simulink model "LQG_non_linear"  (R2022b)
settings: Solver=VariableStepAuto  StartTime=0.0  StopTime=100.0  RelTol=1e-3
values from neighbouring files (symbols this model uses):
  J = get_linearization()    [DK_iteration.m]    (also in LQG.m)
  Kr = lqr(J.A,J.B,Q,R)    [LQG.m]
undefined symbols (not defined in the file or in its folder): a, b, IPy, IPz, Ke, L, rp, std_dev_dx, std_dev_dy, std_dev_phi_dot, std_dev_psi
libraries: simulink x2
settings Model: Creator=alexi  LastModifiedBy=franc

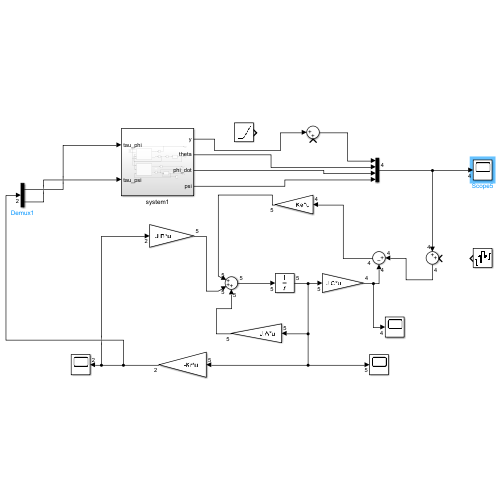
[thumbnail: Simulink's stored preview of the top-level diagram]
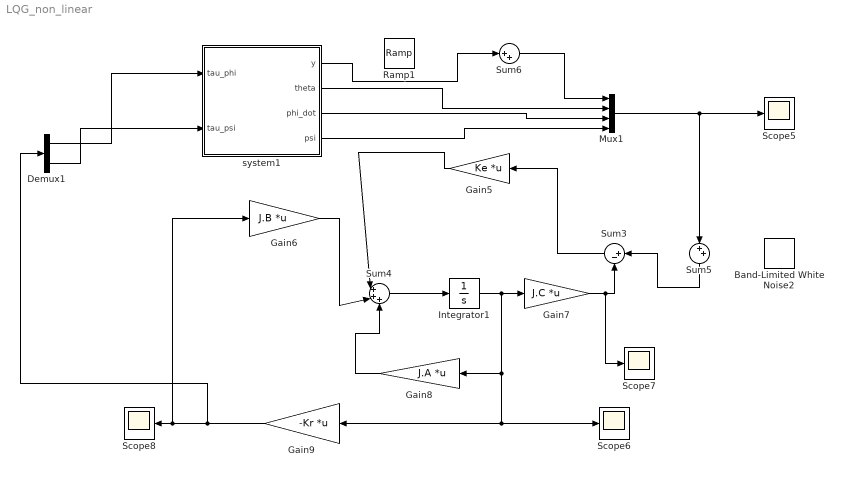
== system LQG_non_linear ==
  Band-Limited White Noise2 : simulink/Sources/Band-Limited White Noise  Cov=[std_dev_dx; std_dev_dy; std_dev_phi_dot; std_dev_psi]  Ts=0.1  seed=[23341]
  Demux1 : Demux  Outputs=2
  Gain5 : Gain  Gain=Ke  Multiplication=Matrix(K*u)
  Gain6 : Gain  Gain=J.B  Multiplication=Matrix(K*u)
  Gain7 : Gain  Gain=J.C  Multiplication=Matrix(K*u)
  Gain8 : Gain  Gain=J.A  Multiplication=Matrix(K*u)
  Gain9 : Gain  Gain=-Kr  Multiplication=Matrix(K*u)
  Integrator1 : Integrator
  Mux1 : Mux
  Ramp1 : simulink/Sources/Ramp  slope=1  start=0  InitialOutput=0
  Scope{5..8} (4 alike) : Scope
  Sum3 : Sum  Inputs=|+-
  Sum4 : Sum  Inputs=|+++
  Sum5 : Sum  Inputs=|++
  Sum6 : Sum  Inputs=|++
  system1 : Subsystem
  wires:
  Gain8/1 -> Sum4/3
  Mux1/1 -> Scope5/1, Sum5/1
  Sum6/1 -> Mux1/1
  Gain5/1 -> Sum4/1
  Gain7/1 -> Scope7/1, Sum3/2
  Sum4/1 -> Integrator1/1
  system1/2(theta) -> Mux1/2
  Sum5/1 -> Sum3/1
  Gain6/1 -> Sum4/2
  Integrator1/1 -> Scope6/1, Gain9/1, Gain8/1, Gain7/1
  Sum3/1 -> Gain5/1
  system1/1(y) -> Sum6/1
  system1/3(phi_dot) -> Mux1/3
  system1/4(psi) -> Mux1/4
  Gain9/1 -> Demux1/1, Gain6/1, Scope8/1
  Demux1/1 -> system1/1(tau_phi)
  Demux1/2 -> system1/2(tau_psi)

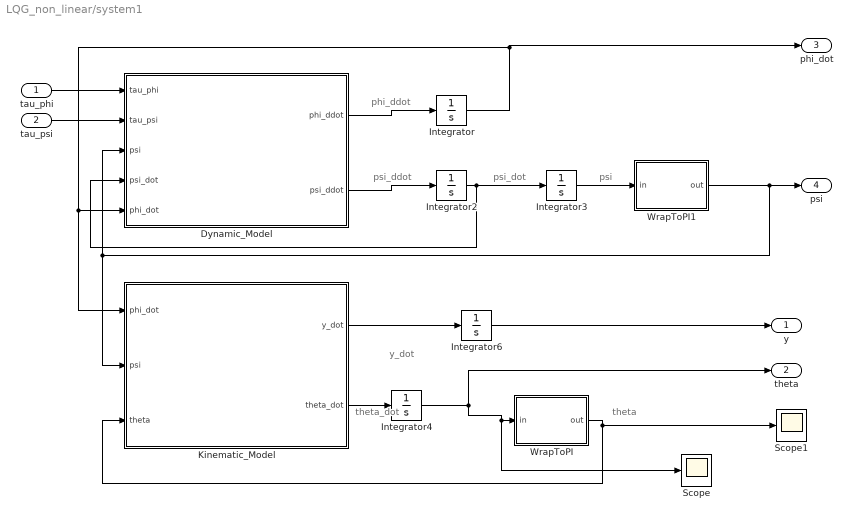
== system LQG_non_linear/system1 ==
  note: theta_dot
  note: psi_dot
  note: psi_ddot
  note: phi_ddot
  note: psi
  note: theta
  note: y_dot
  tau_phi : Inport
  tau_psi : Inport  Port=2
  Dynamic_Model : MATLAB Function  TreatAsAtomicUnit=on
  Integrator : Integrator  InitialCondition=1.1
  Integrator2 : Integrator  InitialCondition=0.1
  Integrator3 : Integrator  InitialCondition=0.1
  Integrator4 : Integrator  InitialCondition=0.1
  Integrator6 : Integrator  InitialCondition=0.2
  Kinematic_Model : MATLAB Function  TreatAsAtomicUnit=on
  Scope : Scope
  Scope1 : Scope
  WrapToPI : MATLAB Function  TreatAsAtomicUnit=on
  WrapToPI1 : MATLAB Function  TreatAsAtomicUnit=on
  y : Outport
  theta : Outport  Port=2
  phi_dot : Outport  Port=3
  psi : Outport  Port=4
  wires:
  Integrator6/1 -> y/1
  WrapToPI1/1(out) -> psi/1, Dynamic_Model/3(psi), Kinematic_Model/2(psi)
  Integrator2/1 -> Integrator3/1, Dynamic_Model/4(psi_dot)
  tau_phi/1 -> Dynamic_Model/1(tau_phi)
  Integrator3/1 -> WrapToPI1/1(in)
  Integrator4/1 -> Scope/1, WrapToPI/1(in), theta/1
  Integrator/1 -> Kinematic_Model/1(phi_dot), Dynamic_Model/5(phi_dot), phi_dot/1
  Kinematic_Model/1(y_dot) -> Integrator6/1
  Kinematic_Model/2(theta_dot) -> Integrator4/1
  Dynamic_Model/2(psi_ddot) -> Integrator2/1
  Dynamic_Model/1(phi_ddot) -> Integrator/1
  WrapToPI/1(out) -> Kinematic_Model/3(theta), Scope1/1
  tau_psi/1 -> Dynamic_Model/2(tau_psi)

== matlab function LQG_non_linear/system1/Dynamic_Model ==
  data: tau_phi input; tau_psi input; phi_ddot output; psi input; psi_dot input; phi_dot input; psi_ddot output; IPz parameter; IPy parameter; L parameter; rp parameter; b parameter; a parameter
function [phi_ddot,psi_ddot] = DynamicModel(tau_phi,tau_psi,psi,psi_dot,phi_dot,IPz, IPy, L, rp, b, a)
    B = [a*rp^2*cos(psi)^2+b*(rp/L)^2*sin(psi)^2+IPy, -IPz*(rp/L)*sin(psi)
        -IPz*(rp/L)*sin(psi), IPz];
    
    C = [(rp^2*b/L^2-a*rp^2)*cos(psi)*sin(psi)*psi_dot*phi_dot;
            -IPz*rp/L*cos(psi)*psi_dot*phi_dot];

    tau = [tau_phi;
            tau_psi];

    q_ddot = inv(B) * (tau - C);

    phi_ddot = q_ddot(1,:);
    psi_ddot = q_ddot(2,:);

== matlab function LQG_non_linear/system1/Kinematic_Model ==
  data: phi_dot input; psi input; theta input; y_dot output; theta_dot output; rp parameter; L parameter
function [y_dot,theta_dot] = KinematicModel(phi_dot,psi,theta,rp, L)
    x_dot = rp * phi_dot * cos(theta) * cos(psi);
    y_dot = rp * phi_dot * sin(theta) * cos(psi);
    theta_dot = - (rp * phi_dot * sin(psi)) / L;

== matlab function LQG_non_linear/system1/WrapToPI ==
  data: in input; out output
function out = wrapper(in)
    out = wrapTo2Pi(in);

== matlab function LQG_non_linear/system1/WrapToPI1 ==
  data: in input; out output
function out = wrapper(in)
    out = wrapToPi(in);
